simulink model "pcc_actuator_to_configuration_mapping_identification"  (R2021a)
settings: Solver=VariableStepAuto  StartTime=0.0  StopTime=10  RelTol=1e-3
values from neighbouring files (symbols this model uses):
  l = out.l.Data    [animate_pcc.m]    (also in config.m = 0.110*[1;1;1])
  s_step_gain = s    [identify_actuator_to_configuration_mapping.m]
undefined symbols (not defined in the file or in its folder): mu_p_eq, tol_q_stable
libraries: simulink x3, simulink_extras x3
settings Model: PauseTimes=0  Creator=maximilianstoelzle  LastModifiedBy=mstolzle
settings RTWCC: BuildConfiguration=Faster Runs

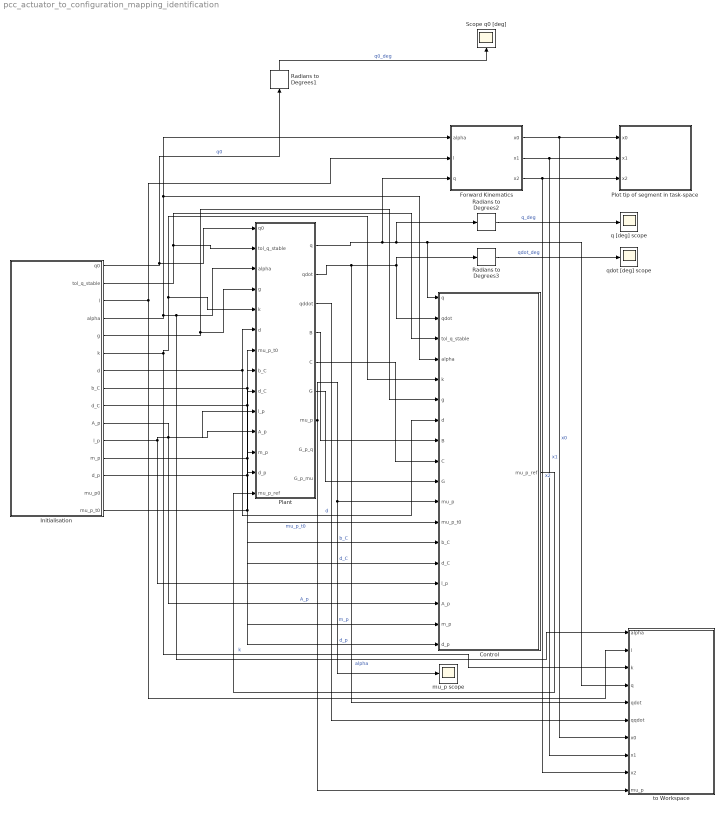
== system pcc_actuator_to_configuration_mapping_identification ==
  Control : Subsystem
  Forward Kinematics : MATLAB Function  TreatAsAtomicUnit=on
  Initialisation : Subsystem
  Plant : Subsystem
  Plot tip of segment in task-space : Subsystem
  Radians to Degrees1 : simulink_extras/Transformations/Radians to Degrees
  Radians to Degrees2 : simulink_extras/Transformations/Radians to Degrees
  Radians to Degrees3 : simulink_extras/Transformations/Radians to Degrees
  Scope q0 [deg] : Scope
  mu_p scope : Scope
  q [deg] scope : Scope
  qdot [deg] scope : Scope
  to Workspace : Subsystem
  wires:
  Plant/3(qddot) -> to Workspace/6(qqdot)
  Initialisation/12(m_p) -> Plant/12(m_p), Control/17(m_p)  "m_p"
  Initialisation/3(l) -> Forward Kinematics/2(l), to Workspace/2(l)
  Radians to Degrees2/1 -> q [deg] scope/1  "q_deg"
  Initialisation/11(l_p) -> Plant/10(l_p), Control/15(l_p)
  Initialisation/1(q0) -> Radians to Degrees1/1, Plant/1(q0)  "q0"
  Forward Kinematics/3(x2) -> to Workspace/9(x2), Plot tip of segment in task-space/3(x2)  "x2"
  Plant/6(G) -> Control/10(G)
  Plant/4(B) -> Control/8(B)
  Initialisation/6(k) -> Control/5(k), Plant/5(k), to Workspace/3(k)  "k"
  Radians to Degrees3/1 -> qdot [deg] scope/1  "qdot_deg"
  Radians to Degrees1/1 -> Scope q0 [deg]/1  "q0_deg"
  Initialisation/2(tol_q_stable) -> Plant/2(tol_q_stable), Control/3(tol_q_stable)
  Plant/5(C) -> Control/9(C)
  Initialisation/13(d_p) -> Plant/13(d_p), Control/18(d_p)  "d_p"
  Initialisation/5(g) -> Plant/4(g), Control/6(g)
  Initialisation/4(alpha) -> to Workspace/1(alpha), Plant/3(alpha), Forward Kinematics/1(alpha), Control/4(alpha)  "alpha"
  Initialisation/7(d) -> Plant/6(d), Control/7(d)  "d"
  Plant/2(qdot) -> Control/2(qdot), Radians to Degrees3/1, to Workspace/5(qdot)
  Plant/1(q) -> Control/1(q), to Workspace/4(q), Radians to Degrees2/1, Forward Kinematics/3(q)
  Initialisation/10(A_p) -> Plant/11(A_p), Control/16(A_p)  "A_p"
  Initialisation/9(d_C) -> Plant/9(d_C), Control/14(d_C)  "d_C"
  Initialisation/8(b_C) -> Plant/8(b_C), Control/13(b_C)  "b_C"
  Plant/7(mu_p) -> mu_p scope/1, Control/11(mu_p), to Workspace/10(mu_p)
  Forward Kinematics/1(x0) -> to Workspace/7(x0), Plot tip of segment in task-space/1(x0)  "x0"
  Forward Kinematics/2(x1) -> to Workspace/8(x1), Plot tip of segment in task-space/2(x1)  "x1"
  Initialisation/15(mu_p_t0) -> Plant/7(mu_p_t0), Control/12(mu_p_t0)  "mu_p_t0"
  Control/1(mu_p_ref) -> Plant/14(mu_p_ref)

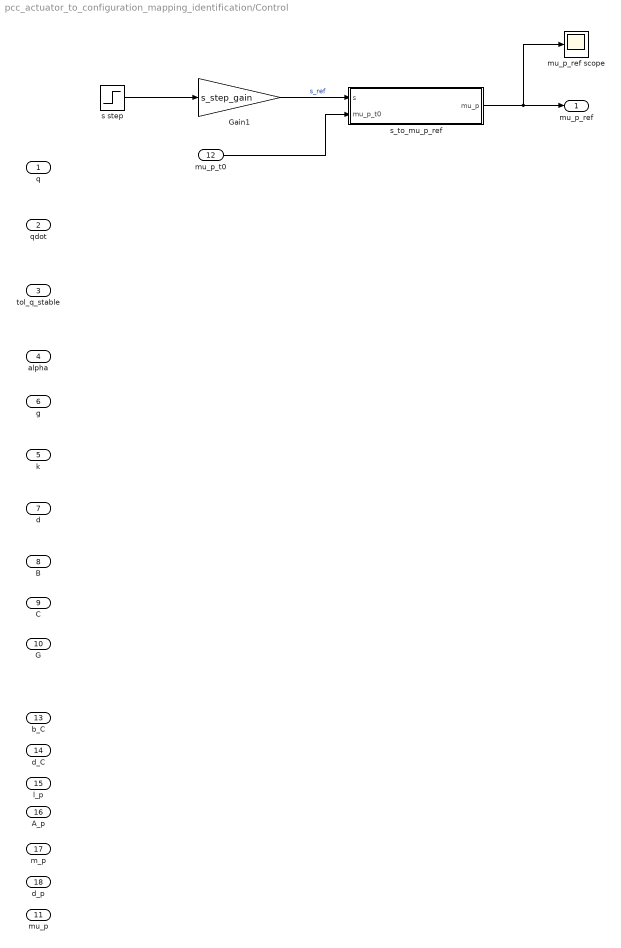
== system pcc_actuator_to_configuration_mapping_identification/Control ==
  q : Inport
  qdot : Inport  Port=2
  tol_q_stable : Inport  Port=3
  alpha : Inport  Port=4
  k : Inport  Port=5
  g : Inport  Port=6
  d : Inport  Port=7
  B : Inport  Port=8
  C : Inport  Port=9
  G : Inport  Port=10
  mu_p : Inport  Port=11
  mu_p_t0 : Inport  Port=12
  b_C : Inport  Port=13
  d_C : Inport  Port=14
  l_p : Inport  Port=15
  A_p : Inport  Port=16
  m_p : Inport  Port=17
  d_p : Inport  Port=18
  Gain1 : Gain  Gain=s_step_gain
  mu_p_ref scope : Scope
  s step : Step  SampleTime=2
  s_to_mu_p_ref : MATLAB Function  TreatAsAtomicUnit=on
  mu_p_ref : Outport
  wires:
  s step/1 -> Gain1/1
  Gain1/1 -> s_to_mu_p_ref/1(s)  "s_ref"
  mu_p_t0/1 -> s_to_mu_p_ref/2(mu_p_t0)
  s_to_mu_p_ref/1(mu_p) -> mu_p_ref scope/1, mu_p_ref/1

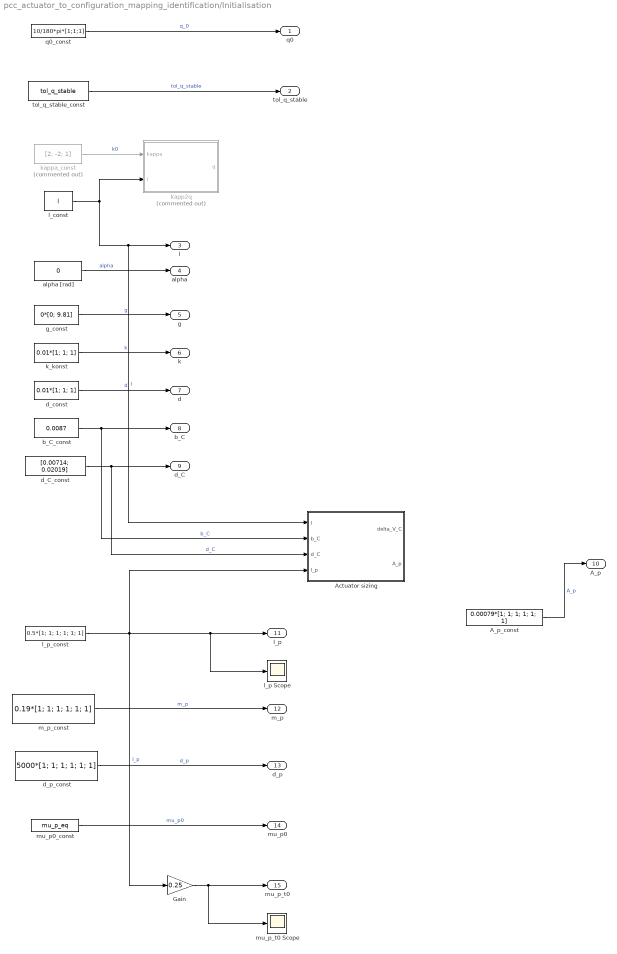
== system pcc_actuator_to_configuration_mapping_identification/Initialisation ==
  A_p_const : Constant  Value=0.00079*[1; 1; 1; 1; 1; 1]
  Actuator sizing : MATLAB Function  TreatAsAtomicUnit=on
  Gain : Gain  Gain=0.25
  alpha [rad] : Constant  Value=0
  b_C_const : Constant  Value=0.0087
  d_C_const : Constant  Value=[0.00714; 0.02019]
  d_const : Constant  Value=0.01*[1; 1; 1]
  d_p_const : Constant  Value=5000*[1; 1; 1; 1; 1; 1]
  g_const : Constant  Value=0*[0; 9.81]
  k_konst : Constant  Value=0.01*[1; 1; 1]
  kapp2q : MATLAB Function  Commented=on  TreatAsAtomicUnit=on
  kappa_const : Constant  Commented=on  Value=[2; -2; 1]
  l_const : Constant  Value=l
  l_p Scope : Scope
  l_p_const : Constant  Value=0.5*[1; 1; 1; 1; 1; 1]
  m_p_const : Constant  Value=0.19*[1; 1; 1; 1; 1; 1]
  mu_p0_const : Constant  Value=mu_p_eq
  mu_p_t0 Scope : Scope
  q0_const : Constant  Value=10/180*pi*[1;1;1]
  tol_q_stable_const : Constant  Value=tol_q_stable
  q0 : Outport
  tol_q_stable : Outport  Port=2
  l : Outport  Port=3
  alpha : Outport  Port=4
  g : Outport  Port=5
  k : Outport  Port=6
  d : Outport  Port=7
  b_C : Outport  Port=8
  d_C : Outport  Port=9
  A_p : Outport  Port=10
  l_p : Outport  Port=11
  m_p : Outport  Port=12
  d_p : Outport  Port=13
  mu_p0 : Outport  Port=14
  mu_p_t0 : Outport  Port=15
  wires:
  kappa_const/1 -> kapp2q/1(kappa)  "k0"
  l_const/1 -> Actuator sizing/1(l), l/1, kapp2q/2(l)  "l"
  alpha [rad]/1 -> alpha/1  "alpha"
  g_const/1 -> g/1  "g"
  k_konst/1 -> k/1  "k"
  d_C_const/1 -> Actuator sizing/3(d_C), d_C/1  "d_C"
  m_p_const/1 -> m_p/1  "m_p"
  b_C_const/1 -> Actuator sizing/2(b_C), b_C/1  "b_C"
  l_p_const/1 -> Gain/1, Actuator sizing/4(l_p), l_p Scope/1, l_p/1  "l_p"
  Gain/1 -> mu_p_t0 Scope/1, mu_p_t0/1
  d_const/1 -> d/1  "d"
  A_p_const/1 -> A_p/1  "A_p"
  q0_const/1 -> q0/1  "q_0"
  tol_q_stable_const/1 -> tol_q_stable/1  "tol_q_stable"
  mu_p0_const/1 -> mu_p0/1  "mu_p0"
  d_p_const/1 -> d_p/1  "d_p"

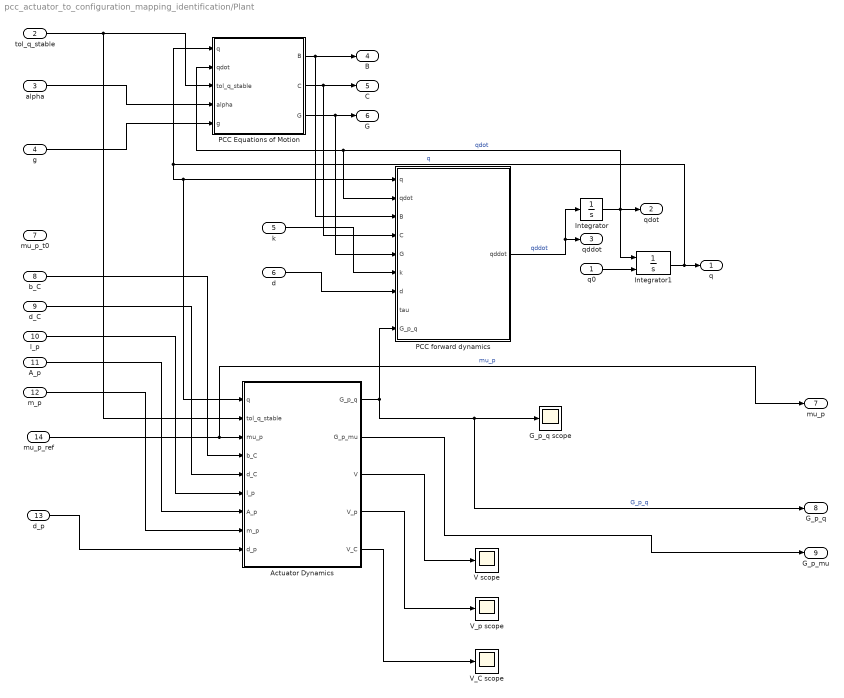
== system pcc_actuator_to_configuration_mapping_identification/Plant ==
  q0 : Inport
  tol_q_stable : Inport  Port=2
  alpha : Inport  Port=3
  g : Inport  Port=4
  k : Inport  Port=5
  d : Inport  Port=6
  mu_p_t0 : Inport  Port=7
  b_C : Inport  Port=8
  d_C : Inport  Port=9
  l_p : Inport  Port=10
  A_p : Inport  Port=11
  m_p : Inport  Port=12
  d_p : Inport  Port=13
  mu_p_ref : Inport  Port=14
  Actuator Dynamics : MATLAB Function  TreatAsAtomicUnit=on
  G_p_q scope : Scope
  Integrator : Integrator  InitialCondition=[0; 0; 0]
  Integrator1 : Integrator  InitialConditionSource=external
  PCC Equations of Motion : MATLAB Function  TreatAsAtomicUnit=on
  PCC forward dynamics : MATLAB Function  TreatAsAtomicUnit=on
  V scope : Scope
  V_C scope : Scope
  V_p scope : Scope
  q : Outport
  qdot : Outport  Port=2
  qddot : Outport  Port=3
  B : Outport  Port=4
  C : Outport  Port=5
  G : Outport  Port=6
  mu_p : Outport  Port=7
  G_p_q : Outport  Port=8
  G_p_mu : Outport  Port=9
  wires:
  g/1 -> PCC Equations of Motion/5(g)
  alpha/1 -> PCC Equations of Motion/4(alpha)
  q0/1 -> Integrator1/2
  k/1 -> PCC forward dynamics/6(k)
  PCC Equations of Motion/3(G) -> PCC forward dynamics/5(G), G/1
  PCC Equations of Motion/1(B) -> PCC forward dynamics/3(B), B/1
  Integrator1/1 -> PCC Equations of Motion/1(q), PCC forward dynamics/1(q), Actuator Dynamics/1(q), q/1  "q"
  PCC forward dynamics/1(qddot) -> Integrator/1, qddot/1  "qddot"
  d/1 -> PCC forward dynamics/7(d)
  Integrator/1 -> PCC forward dynamics/2(qdot), PCC Equations of Motion/2(qdot), Integrator1/1, qdot/1  "qdot"
  PCC Equations of Motion/2(C) -> PCC forward dynamics/4(C), C/1
  A_p/1 -> Actuator Dynamics/7(A_p)
  m_p/1 -> Actuator Dynamics/8(m_p)
  d_C/1 -> Actuator Dynamics/5(d_C)
  b_C/1 -> Actuator Dynamics/4(b_C)
  l_p/1 -> Actuator Dynamics/6(l_p)
  mu_p_ref/1 -> mu_p/1, Actuator Dynamics/3(mu_p)  "mu_p"
  Actuator Dynamics/1(G_p_q) -> PCC forward dynamics/9(G_p_q), G_p_q scope/1, G_p_q/1  "G_p_q"
  Actuator Dynamics/2(G_p_mu) -> G_p_mu/1
  Actuator Dynamics/3(V) -> V scope/1
  Actuator Dynamics/5(V_C) -> V_C scope/1
  Actuator Dynamics/4(V_p) -> V_p scope/1
  tol_q_stable/1 -> Actuator Dynamics/2(tol_q_stable), PCC Equations of Motion/3(tol_q_stable)
  d_p/1 -> Actuator Dynamics/9(d_p)

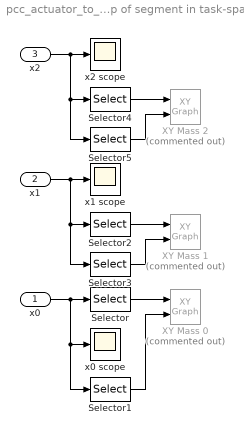
== system pcc_actuator_to_configuration_mapping_identification/Plot tip of segment in task-space ==
  x0 : Inport
  x1 : Inport  Port=2
  x2 : Inport  Port=3
  Selector : Selector  InputPortWidth=2  IndexOptions=Index vector (dialog)  Indices=[1]  OutputSizes=1
  Selector1 : Selector  InputPortWidth=2  IndexOptions=Index vector (dialog)  Indices=[2]  OutputSizes=1
  Selector2 : Selector  InputPortWidth=2  IndexOptions=Index vector (dialog)  Indices=[1]  OutputSizes=1
  Selector3 : Selector  InputPortWidth=2  IndexOptions=Index vector (dialog)  Indices=[2]  OutputSizes=1
  Selector4 : Selector  InputPortWidth=2  IndexOptions=Index vector (dialog)  Indices=[1]  OutputSizes=1
  Selector5 : Selector  InputPortWidth=2  IndexOptions=Index vector (dialog)  Indices=[2]  OutputSizes=1
  XY Mass 0 : simulink/Sinks/XY Graph  Commented=on  xmin=-1.2*sum(l)  xmax=1.2*sum(l)  ymin=-1.2*sum(l)  ymax=1.2*sum(l)  st=-1
  XY Mass 1 : simulink/Sinks/XY Graph  Commented=on  xmin=-1.2*sum(l)  xmax=1.2*sum(l)  ymin=-1.2*sum(l)  ymax=1.2*sum(l)  st=-1
  XY Mass 2 : simulink/Sinks/XY Graph  Commented=on  xmin=-1.2*sum(l)  xmax=1.2*sum(l)  ymin=-1.2*sum(l)  ymax=1.2*sum(l)  st=-1
  x0 scope : Scope
  x1 scope : Scope
  x2 scope : Scope
  wires:
  x2/1 -> Selector5/1, Selector4/1, x2 scope/1
  Selector/1 -> XY Mass 0/1
  x1/1 -> Selector3/1, Selector2/1, x1 scope/1
  Selector5/1 -> XY Mass 2/2
  Selector3/1 -> XY Mass 1/2
  Selector1/1 -> XY Mass 0/2
  x0/1 -> x0 scope/1, Selector1/1, Selector/1
  Selector4/1 -> XY Mass 2/1
  Selector2/1 -> XY Mass 1/1

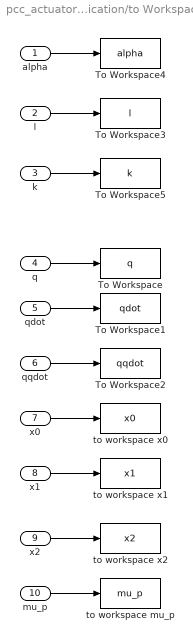
== system pcc_actuator_to_configuration_mapping_identification/to Workspace ==
  alpha : Inport
  l : Inport  Port=2
  k : Inport  Port=3
  q : Inport  Port=4
  qdot : Inport  Port=5
  qqdot : Inport  Port=6
  x0 : Inport  Port=7
  x1 : Inport  Port=8
  x2 : Inport  Port=9
  mu_p : Inport  Port=10
  To Workspace : ToWorkspace  VariableName=q  SaveFormat=Timeseries  SampleTime=-1
  To Workspace1 : ToWorkspace  VariableName=qdot  SaveFormat=Timeseries  SampleTime=-1
  To Workspace2 : ToWorkspace  VariableName=qqdot  SaveFormat=Timeseries  SampleTime=-1
  To Workspace3 : ToWorkspace  VariableName=l  SaveFormat=Timeseries  SampleTime=-1
  To Workspace4 : ToWorkspace  VariableName=alpha  SaveFormat=Timeseries  SampleTime=-1
  To Workspace5 : ToWorkspace  VariableName=k  SaveFormat=Timeseries  SampleTime=-1
  to workspace mu_p : ToWorkspace  VariableName=mu_p  SaveFormat=Timeseries  SampleTime=-1
  to workspace x0 : ToWorkspace  VariableName=x0  SaveFormat=Timeseries  SampleTime=-1
  to workspace x1 : ToWorkspace  VariableName=x1  SaveFormat=Timeseries  SampleTime=-1
  to workspace x2 : ToWorkspace  VariableName=x2  SaveFormat=Timeseries  SampleTime=-1
  wires:
  alpha/1 -> To Workspace4/1
  qdot/1 -> To Workspace1/1
  l/1 -> To Workspace3/1
  qqdot/1 -> To Workspace2/1
  q/1 -> To Workspace/1
  mu_p/1 -> to workspace mu_p/1
  x0/1 -> to workspace x0/1
  x1/1 -> to workspace x1/1
  x2/1 -> to workspace x2/1
  k/1 -> To Workspace5/1

== matlab function pcc_actuator_to_configuration_mapping_identification/Initialisation/Actuator sizing ==
  data: l input; delta_V_C output; b_C input; d_C input; l_p input; A_p output
function [delta_V_C, A_p]= piston_sizing(l, b_C, d_C, l_p)
    q_min = -90/180*pi*ones(length(l), 1);
    q_max = 90/180*pi*ones(length(l), 1);
    delta_V_C = abs(V_C_fun(q_max, b_C, d_C) - V_C_fun(q_min, b_C, d_C));
    A_p = 1*delta_V_C ./ l_p;
end

== matlab function pcc_actuator_to_configuration_mapping_identification/Forward Kinematics ==
  data: alpha input; l input; x0 output; q input; x1 output; x2 output
function [x0, x1, x2] = forward_kinematics(alpha, l, q)
    % introduce tolerance for numerical stability
    q = set_min_abs_val(q, 0.005);

    x0 = q2x0_fun(l(1), q, alpha);
    x1 = q2x1_fun(l(2), q, alpha);
    x2 = q2x2_fun(l(3), q, alpha);
end

== matlab function pcc_actuator_to_configuration_mapping_identification/Plant/PCC forward dynamics ==
  data: q input; qdot input; B input; qddot output; C input; G input; k input; d input; tau input; G_p_q input
function qddot  = pcc_forward_dynamics(q, qdot, B, C, G, k, d, tau, G_p_q)
   qddot = B^(-1)*(-(C*qdot)-G-(k.*q)-(d.*qdot)-G_p_q+tau);
end

== matlab function pcc_actuator_to_configuration_mapping_identification/Initialisation/kapp2q ==
  data: kappa input; q output; l input
function q = kappa2q(kappa, l)
    q = [kappa(1) * l(1);
         kappa(2) * l(2);
         kappa(3) * l(3)];
end

== matlab function pcc_actuator_to_configuration_mapping_identification/Plant/PCC Equations of Motion ==
  data: q input; qdot input; tol_q_stable input; alpha input; B output; g input; C output; G output
function [B, C, G]  = pcc_eom(q, qdot, tol_q_stable, alpha, g)
    % introduce tolerance for numerical stability
    q_stable = set_min_abs_val(q, tol_q_stable);
    
    B = B_fun(q_stable);
    
    C = C_fun(q_stable, qdot);
    
    G = G_fun(q_stable, alpha, g);
end

== matlab function pcc_actuator_to_configuration_mapping_identification/Control/s_to_mu_p_ref ==
  data: s input; mu_p output; mu_p_t0 input
function mu_p = s_to_mu_p(s, mu_p_t0)
    mu_p = zeros(2*length(s), 1);
    % s1 = mu_p1 - mu_p2
    % q > 0 --> p2 > p1 --> V_p1 > V_p2 --> mu_p1 > mu_p2 --> s1 > 0
    for i = 1:length(s)
       mu_p(2*i - 1) = mu_p_t0(2*i - 1) + s(i) / 2;
       mu_p(2*i) = mu_p_t0(2*i) - s(i) / 2;
    end
end

== matlab function pcc_actuator_to_configuration_mapping_identification/Plant/Actuator Dynamics ==
  data: q input; tol_q_stable input; mu_p input; b_C input; d_C input; l_p input; A_p input; G_p_q output; G_p_mu output; m_p input; d_p input; V output; V_p output; V_C output
function [G_p_q, G_p_mu, V, V_p, V_C]  = actuator_dynamics(q, tol_q_stable, mu_p, b_C, d_C, l_p, A_p, m_p, d_p)
    % introduce tolerance for numerical stability
    q_stable = set_min_abs_val(q, tol_q_stable);

    % volume of fluid
    V = V_fun(q_stable, mu_p, A_p, b_C, d_C);
    V_p = V_p_fun(mu_p, A_p);
    V_C = V_C_fun(q_stable, b_C, d_C);

    % potential forces by fluid
    G_p_q = G_p_q_fun(q_stable, mu_p, l_p, A_p, b_C, d_C);
    G_p_mu = G_p_mu_fun(q_stable, mu_p, l_p, A_p, b_C, d_C);
end
